simulink model "DK_truot"  (R2023a)
settings: Solver=ode4  StartTime=0.0  StopTime=50  FixedStep=0.001  RelTol=1e-3
settings Model: Creator=VINH  LastModifiedBy=VINH

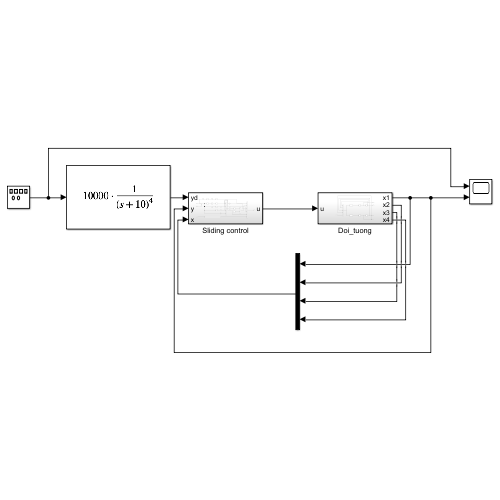
[thumbnail: Simulink's stored preview of the top-level diagram]
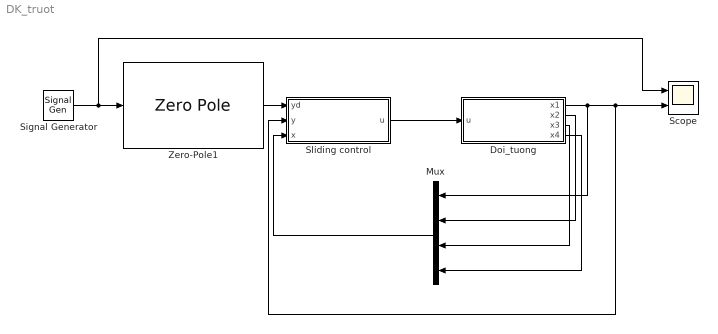
== system DK_truot ==
  Doi_tuong : Subsystem
  Mux : Mux
  Scope : Scope  NumInputPorts=2
  Signal Generator : SignalGenerator  Amplitude=0.5  Frequency=0.1
  Sliding control : Subsystem
  Zero-Pole1 : ZeroPole  Zeros=[]  Poles=[-10 -10 -10 -10]  Gain=10000
  wires:
  Sliding control/1(u) -> Doi_tuong/1(u)
  Doi_tuong/1(x1) -> Mux/1, Scope/2, Sliding control/2(y)
  Doi_tuong/2(x2) -> Mux/2
  Doi_tuong/3(x3) -> Mux/3
  Doi_tuong/4(x4) -> Mux/4
  Mux/1 -> Sliding control/3(x)
  Signal Generator/1 -> Zero-Pole1/1, Scope/1
  Zero-Pole1/1 -> Sliding control/1(yd)

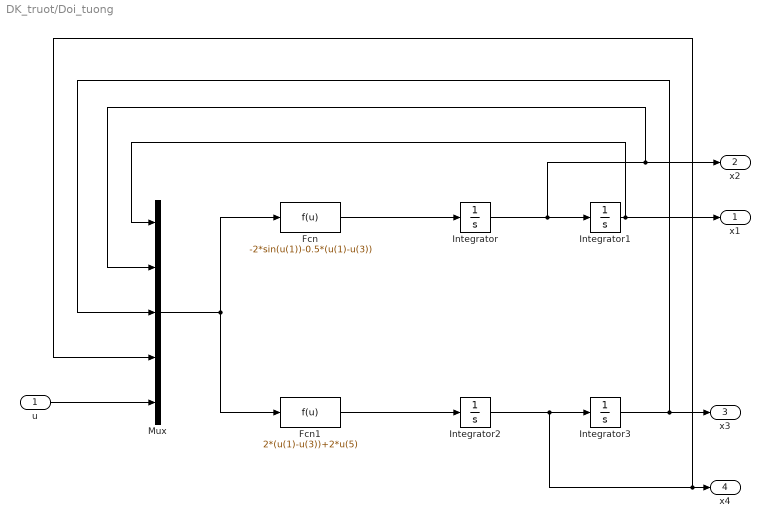
== system DK_truot/Doi_tuong ==
  u : Inport
  Fcn : Fcn  Expr=-2*sin(u(1))-0.5*(u(1)-u(3))
  Fcn1 : Fcn  Expr=2*(u(1)-u(3))+2*u(5)
  Integrator{,1..3} (4 alike) : Integrator
  Mux : Mux  Inputs=5
  x1 : Outport
  x2 : Outport  Port=2
  x3 : Outport  Port=3
  x4 : Outport  Port=4
  wires:
  Mux/1 -> Fcn1/1, Fcn/1
  Fcn/1 -> Integrator/1
  Integrator/1 -> Mux/2, x2/1, Integrator1/1
  Fcn1/1 -> Integrator2/1
  Integrator2/1 -> Mux/4, x4/1, Integrator3/1
  Integrator1/1 -> Mux/1, x1/1
  Integrator3/1 -> Mux/3, x3/1
  u/1 -> Mux/5

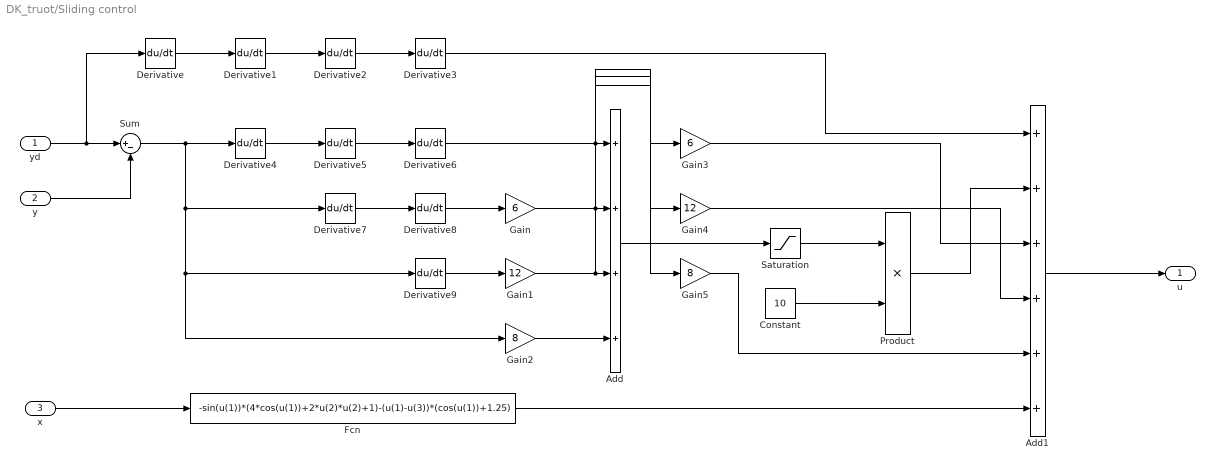
== system DK_truot/Sliding control ==
  yd : Inport
  y : Inport  Port=2
  x : Inport  Port=3
  Add : Sum  Inputs=++++
  Add1 : Sum  Inputs=++++++
  Constant : Constant  Value=10
  Derivative{,1..9} (10 alike) : Derivative
  Fcn : Fcn  Expr=-sin(u(1))*(4*cos(u(1))+2*u(2)*u(2)+1)-(u(1)-u(3))*(cos(u(1))+1.25)
  Gain : Gain  Gain=6
  Gain1 : Gain  Gain=12
  Gain2 : Gain  Gain=8
  Gain3 : Gain  Gain=6
  Gain4 : Gain  Gain=12
  Gain5 : Gain  Gain=8
  Product : Product
  Saturation : Saturate  UpperLimit=2  LowerLimit=-2
  Sum : Sum  Inputs=|+-
  u : Outport
  wires:
  yd/1 -> Sum/1, Derivative/1
  y/1 -> Sum/2
  Derivative/1 -> Derivative1/1
  Derivative1/1 -> Derivative2/1
  Derivative2/1 -> Derivative3/1
  Sum/1 -> Derivative4/1, Derivative7/1, Derivative9/1, Gain2/1
  Derivative4/1 -> Derivative5/1
  Derivative5/1 -> Derivative6/1
  Derivative7/1 -> Derivative8/1
  Derivative8/1 -> Gain/1
  Derivative9/1 -> Gain1/1
  Derivative6/1 -> Gain3/1, Add/1
  Gain/1 -> Gain4/1, Add/2
  Gain1/1 -> Gain5/1, Add/3
  Gain2/1 -> Add/4
  Add/1 -> Saturation/1
  Saturation/1 -> Product/1
  Constant/1 -> Product/2
  x/1 -> Fcn/1
  Fcn/1 -> Add1/6
  Derivative3/1 -> Add1/1
  Product/1 -> Add1/2
  Gain3/1 -> Add1/3
  Gain4/1 -> Add1/4
  Gain5/1 -> Add1/5
  Add1/1 -> u/1
